simulink model "simplePendulumOnACart0"  (R2023a)
settings: Solver=VariableStepAuto  StartTime=0.0  StopTime=50  FixedStep=0.00002  RelTol=1e-3
values from neighbouring files (symbols this model uses):
  accel_gravity = 10    [simplePendulumOnACart_v0.m]
  C = [1 0 0 0]    [simplePendulumOnACart_v0.m]
  cart_mass = 2    [simplePendulumOnACart_v0.m]
  error_q0 = -q0    (= 0)    [simplePendulumOnACart_v0.m]
  F = (place(A_0', -C', 5*[-10 -10.01 -40.02 -20.03]))'    [simplePendulumOnACart_v0.m]
  initial_condition = [q0; qdot0; theta0; thetadot0]    [simplePendulumOnACart_v0.m]
  Ka_pair = [Ka_pi_destabilize; Ka_0_stabilize]    [simplePendulumOnACart_v0.m]
  lin_spring_stiff = 0    [simplePendulumOnACart_v0.m]
  pendulum_length = l    [animate_pendulum_cart.m]    (also in simplePendulumOnACart_v0.m = 0.3)
  pendulum_mass = 1    [simplePendulumOnACart_v0.m]
  rot_spring_stiff = 0    [simplePendulumOnACart_v0.m]
  up = 1    [simplePendulumOnACart_v0.m]
  x_eq_down = [q_eq; 0; 0; 0]    [simplePendulumOnACart_v0.m]
  x_eq_up = [q_eq; 0; pi; 0]    [simplePendulumOnACart_v0.m]
settings Model: Creator=sagar  LastModifiedBy=sagar

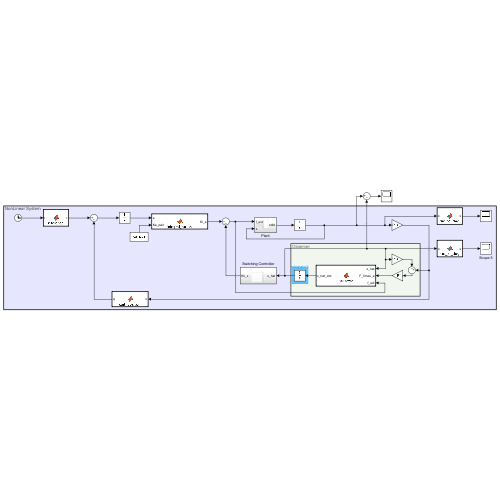
[thumbnail: Simulink's stored preview of the top-level diagram]
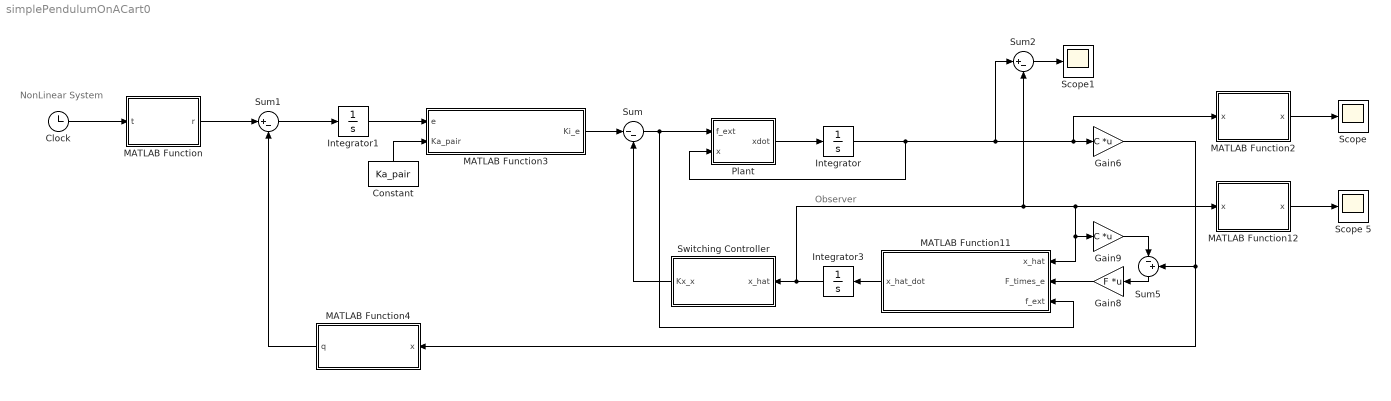
== system simplePendulumOnACart0 ==
  note: Observer
  note: NonLinear System
  Clock : Clock
  Constant : Constant  Value=Ka_pair
  Gain6 : Gain  Gain=C  Multiplication=Matrix(K*u)
  Gain8 : Gain  Gain=F  Multiplication=Matrix(K*u)
  Gain9 : Gain  Gain=C  Multiplication=Matrix(K*u)
  Integrator : Integrator  InitialCondition=initial_condition
  Integrator1 : Integrator  InitialCondition=error_q0
  Integrator3 : Integrator  InitialCondition=initial_condition
  MATLAB Function : MATLAB Function  TreatAsAtomicUnit=on
  MATLAB Function11 : MATLAB Function  TreatAsAtomicUnit=on
  MATLAB Function12 : MATLAB Function  TreatAsAtomicUnit=on
  MATLAB Function2 : MATLAB Function  TreatAsAtomicUnit=on
  MATLAB Function3 : MATLAB Function  TreatAsAtomicUnit=on
  MATLAB Function4 : MATLAB Function  TreatAsAtomicUnit=on
  Plant : Subsystem
  Scope : Scope
  Scope 5 : Scope
  Scope1 : Scope
  Sum : Sum  Inputs=|--
  Sum1 : Sum  Inputs=|+-
  Sum2 : Sum  Inputs=|+-
  Sum5 : Sum  Inputs=|-+
  Switching Controller : Subsystem
  wires:
  Clock/1 -> MATLAB Function/1(t)
  MATLAB Function2/1(x) -> Scope/1
  Integrator/1 -> Plant/2(x), Sum2/1, MATLAB Function2/1("x "), Gain6/1
  Switching Controller/1(Kx_x) -> Sum/2
  Integrator1/1 -> MATLAB Function3/1(e)
  MATLAB Function3/1(Ki_e) -> Sum/1
  Constant/1 -> MATLAB Function3/2(Ka_pair)
  Sum1/1 -> Integrator1/1
  MATLAB Function/1(r) -> Sum1/1
  MATLAB Function4/1(q) -> Sum1/2
  Sum/1 -> Plant/1(f_ext), MATLAB Function11/3(f_ext)
  Plant/1(xdot) -> Integrator/1
  Gain6/1 -> MATLAB Function4/1(x), Sum5/2
  MATLAB Function11/1(x_hat_dot) -> Integrator3/1
  Integrator3/1 -> MATLAB Function11/1(x_hat), Gain9/1, MATLAB Function12/1("x "), Sum2/2, Switching Controller/1(x_hat)
  Gain8/1 -> MATLAB Function11/2(F_times_e)
  Sum5/1 -> Gain8/1
  Gain9/1 -> Sum5/1
  MATLAB Function12/1(x) -> Scope 5/1
  Sum2/1 -> Scope1/1

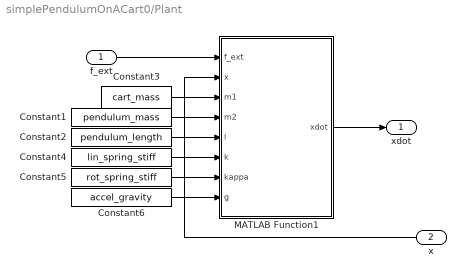
== system simplePendulumOnACart0/Plant ==
  f_ext : Inport
  x : Inport  Port=2
  Constant1 : Constant  Value=pendulum_mass
  Constant2 : Constant  Value=pendulum_length
  Constant3 : Constant  Value=cart_mass
  Constant4 : Constant  Value=lin_spring_stiff
  Constant5 : Constant  Value=rot_spring_stiff
  Constant6 : Constant  Value=accel_gravity
  MATLAB Function1 : MATLAB Function  TreatAsAtomicUnit=on
  xdot : Outport
  wires:
  Constant6/1 -> MATLAB Function1/8(g)
  MATLAB Function1/1(xdot) -> xdot/1
  Constant2/1 -> MATLAB Function1/5(l)
  x/1 -> MATLAB Function1/2(x)
  Constant5/1 -> MATLAB Function1/7(kappa)
  Constant1/1 -> MATLAB Function1/4(m2)
  Constant3/1 -> MATLAB Function1/3(m1)
  Constant4/1 -> MATLAB Function1/6(k)
  f_ext/1 -> MATLAB Function1/1(f_ext)

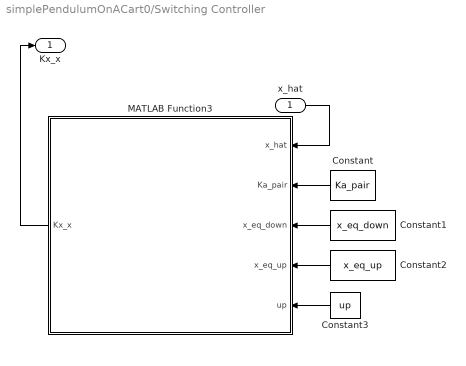
== system simplePendulumOnACart0/Switching Controller ==
  x_hat : Inport
  Constant : Constant  Value=Ka_pair
  Constant1 : Constant  Value=x_eq_down
  Constant2 : Constant  Value=x_eq_up
  Constant3 : Constant  Value=up
  MATLAB Function3 : MATLAB Function  TreatAsAtomicUnit=on
  Kx_x : Outport
  wires:
  x_hat/1 -> MATLAB Function3/1(x_hat)
  Constant/1 -> MATLAB Function3/2(Ka_pair)
  MATLAB Function3/1(Kx_x) -> Kx_x/1
  Constant1/1 -> MATLAB Function3/3(x_eq_down)
  Constant2/1 -> MATLAB Function3/4(x_eq_up)
  Constant3/1 -> MATLAB Function3/5(up)

== matlab function simplePendulumOnACart0/Plant/MATLAB Function1 ==
  data: f_ext input; x input; xdot output; m1 input; m2 input; l input; k input; kappa input; g input
function xdot = pendulum_cart(f_ext, x, m1, m2, l, k, kappa, g)
    % State variables
    q = x(1); qdot = x(2); theta = x(3); thetadot = x(4);

    xdot_1 = qdot;
    xdot_3 = thetadot;
    qddot = (1/(m1 + m2 - m2 * (cos(theta))^2)) *...
            (f_ext + m2 * g * sin(theta) * cos(theta) +...
            (kappa/l) * cos(theta) * theta + k*q +...
             m2 * l * sin(theta) * thetadot^2);
    xdot_2 = qddot;
    xdot_4 = -(cos(theta)/l) * qddot - (g/l) * sin(theta) -...
             (kappa/(m2*(l^2))) * theta;
    xdot = [xdot_1; xdot_2; xdot_3; xdot_4];
end

== matlab function simplePendulumOnACart0/MATLAB Function ==
  data: t input; r output
function r = reference(t)
    if (t < 10)
        r = 0;
    elseif (t < 20)
        r = 5;
    elseif (t < 30)
        r = -2;
    else
        r = 0;
    end
    % r = 0;
end

== matlab function simplePendulumOnACart0/MATLAB Function2 ==
  data: x input; x output
function x = rad_to_deg(x)
    x(3) = rad2deg(x(3));
    x(4) = rad2deg(x(4));
end

== matlab function simplePendulumOnACart0/Switching Controller/MATLAB Function3 ==
  data: x_hat input; Kx_x output; Ka_pair input; x_eq_down input; x_eq_up input; up input
function Kx_x = switching_controller(x_hat, Ka_pair, x_eq_down, x_eq_up, up)
    % States
    q = x_hat(1); qdot = x_hat(2); theta = x_hat(3); thetadot = x_hat(4);

    x_eq = x_eq_down;
    if (3*pi/4 < x_hat(3)) && (x_hat(3) < 5*pi/4) && (up == 1)
        x_eq = x_eq_up;
    end
    del_x = x_hat - x_eq;

    if (up == 1) && (3*pi/4 < theta) && (theta < 5*pi/4)
        Kx_x = Ka_pair(2,1:4) * del_x;
    elseif (up == 1)
        Kx_x = Ka_pair(1,1:4) * del_x;
    elseif (theta == pi)
        Kx_x = Ka_pair(1,1:4) * del_x;
    else
        Kx_x = Ka_pair(2,1:4) * del_x;
    end
end

== matlab function simplePendulumOnACart0/MATLAB Function3 ==
  data: e input; Ki_e output; Ka_pair input
function Ki_e = integral_action(e,Ka_pair)
    Ki_e = e * Ka_pair(2,5);
    % Ki_e = 0;
end

== matlab function simplePendulumOnACart0/MATLAB Function4 ==
  data: x input; q output
function q = cart_position(x)
    q = x(1);
end

== matlab function simplePendulumOnACart0/MATLAB Function11 ==
  data: x_hat input; F_times_e input; f_ext input; x_hat_dot output
function x_hat_dot = observer(x_hat, F_times_e, f_ext)
    % TODO: take m1, m2, l, k, kappa, & g as the input parameters
    m1 = 2; m2 = 1; l = 0.3; k = 0; kappa = 0; g = 10;

    % State variables
    q = x_hat(1); qdot = x_hat(2); theta = x_hat(3); thetadot = x_hat(4);

    qddot = (1/(m1 + m2 - m2 * (cos(theta)^2))) *...
            (f_ext + m2 * g * sin(theta) * cos(theta) -...
            (kappa/l) * cos(theta) * theta + k*q -...
             m2 * l * sin(theta) * thetadot^2);

    thetaddot = -(cos(theta)/l) * qddot - (g/l) * sin(theta) -...
             (kappa/(m2*(l^2))) * theta;
    x_hat_dot = [qdot; qddot; thetadot; thetaddot];
    x_hat_dot = x_hat_dot - F_times_e;
end

== matlab function simplePendulumOnACart0/MATLAB Function12 ==
  data: x input; x output
function x = rad_to_deg(x)
    x(3) = rad2deg(x(3));
    x(4) = rad2deg(x(4));
end
